simulink model "vehicle_motion_model_final_temp"  (R2021b)
settings: Solver=ode5  StartTime=0.0  StopTime=600  FixedStep=0.001  RelTol=1e-3
StopFcn:
  | % stop simulation callback function
  | figure(1);
  | out.x_gt.data = permute(out.x_gt.data,[3, 1, 2]);
  | plot3(out.x_gt.data(:, 1), out.x_gt.data(:, 2), -out.x_gt.data(:, 3), 'Color', 'r', 'LineWidth', 1.5);
  | legend('Истинная траектория')
  | xlabel('X, \itм');
  | ylabel('Y, \itм');
  | zlabel('Z, \itм');
  | figure(2);
  | plot3(out.x.data(:, 1), out.x.data(:, 2), -out.x.data(:, 3), 'Color', 'b', 'LineWidth', 1.5);
  | hold on;
  | xlabel('X, \itм');
  | ylabel('Y, \itм');
  | zlabel('Z, \itм');
  | % legend('pos')
  | hold on;
  | plot3(out.x_gt.data(:, 1), out.x_gt.data(:, 2), -out.x_gt.data(:, 3), 'Color', 'r', 'LineWidth', 1.5);
  | hold on;
  | legend('Рассчитанная траектория', 'Истинная траектория')
  | % errors
  | figure(3);
  | yyaxis left;
  | plot(out.hor_err_fus.time, out.hor_err_fus.data, 'Color', 'b', 'LineWidth', 1.5);
  | xlabel('время, \itс');
  | ylabel('Горизонтальная ошибка, \itм');
  | hold on;
  | yyaxis right;
  | plot(out.ver_err_fus.time, out.ver_err_fus.data, 'Color', 'r', 'LineWidth', 1.5);
  | ylabel('Вертикальная ошибка, \itм');
  | legend('Горизонтальная позиционная ошибка', 'Вертикальная позиционная ошибка');
  | grid on;
  | figure(4);
  | yyaxis left;
  | plot(out.hor_err_ins.time, out.hor_err_ins.data, '-', 'Color', 'b', 'LineWidth', 1.5);
  | xlabel('время, \itс');
  | ylabel('Горизонтальная ошибка, \itм');
  | hold on;
  | yyaxis right;
  | plot(out.ver_err_ins.time, out.ver_err_ins.data, '-', 'Color', 'r', 'LineWidth', 1.5);
  | ylabel('Вертикальная ошибка, \itм');
  | legend('Горизонтальная позиционная ошибка', 'Вертикальная позиционная ошибка');
  | grid on;
model workspace (MAT data in the model file):
  AxlIxx = 62.3745166667
  AxlM = 160
  Cps = 2
  CzWhlAxl = 557955.087061
  DCT_Param : object (value not decoded)
  Downshift_Speeds = [9.5625 12.9375 16.3125 19.6875 23.0625 26.4375 29.8125 33.1875 36.5625 39.9375 43.3125 46.6875 ... (28 elements, 4x7)]
  F0zWhlAxl = 16132.2380068
  HTCH : object (value not decoded)
  Hmax = 0.25
  KzWhlAxl = 58428920.0848
  NCyl = 6
  Pedal_Positions = [0.1 0.4 0.5 0.9]
  Pstd = 101325
  Q = [1  0  0; 0  1  0; 0  0  1]
  Rair = 287
  SUS : object (value not decoded)
  TRA : object (value not decoded)
  Trans : object (value not decoded)
  Tstd = 293.15
  Upshift_Speeds = [12.9375 16.3125 19.6875 33 26.4375 29.8125 33.1875 52.5 39.9375 43.3125 46.6875 77.25 ... (28 elements, 4x7)]
  VEH : object (value not decoded)
  Vd = 0.00346
  WH : Mass (value not decoded)
  dt3D = 0.05
  f_air = [0 0 0 0 0 0 0 0 0 0 0 0 ... (256 elements, 16x16)]
  f_co = [0 0 0 0 0 0 0 0 0 0 0 0 ... (256 elements, 16x16)]
  f_co2 = [0 0 0 0 0 0 0 0 0 0 0 0 ... (256 elements, 16x16)]
  f_eff = [352.135682859 352.135682859 320.724378192 303.655312657 295.930136708 291.240087194 291.240271258 291.240312459 291.240275452 291.240198499 291.240100781 291.240018769 ... (256 elements, 16x16)]
  f_fuel = [0 0 0 0 0 0 0 0 0 0 0 0 ... (256 elements, 16x16)]
  f_hc = [0 0 0 0 0 0 0 0 0 0 0 0 ... (256 elements, 16x16)]
  f_nox = [0 0 0 0 0 0 0 0 0 0 0 0 ... (256 elements, 16x16)]
  f_pm = [0 0 0 0 0 0 0 0 0 0 0 0 ... (256 elements, 16x16)]
  f_susp_axl_bp = [1 2]
  f_susp_dz_bp = [-0.325022776267 -0.315022776267 -0.305022776267 -0.205022776267 -0.105022776267 -0.00502277626717 0.0949772237328 0.194977223733 0.204977223733 0.214977223733]
  f_susp_dzdot_bp = [-3 -0.3 -0.2 -0.1 0 0.1 0.2 0.3 3]
  f_susp_fmz = [-144070.391448 -93629.24037 -75929.1118915 -20630.5828179 -15385.48216 -10140.3815021 -4895.28084414 349.819813785 -31916.3973792 18437.6709544 -83996.1993354 -33555.0482577 ... (43920 elements, 10x9x61x2x4)]
  f_susp_geom = [0 0 0 0 0 0 0 0 0 0 0 0 ... (3660 elements, 10x61x2x3)]
  f_susp_strgdelta_bp = [-0.523598775598 -0.506145483078 -0.488692190558 -0.471238898038 -0.453785605519 -0.436332312999 -0.418879020479 -0.401425727959 -0.383972435439 -0.366519142919 -0.349065850399 -0.331612557879 ... (61 elements, 1x61)]
  f_tbrake = [0 76.8593923996 105.140482948 131.533638111 157.926793274 176.658631717 176.65727296 176.656856686 176.656879077 176.657093756 176.657404516 176.65772406 ... (256 elements, 16x16)]
  f_tbrake_n_bpt = [0 649.519052838 912.419621844 1175.32019085 1438.22075986 1701.12132886 1964.02189787 2226.92246687 2489.82303588 2752.72360489 3015.62417389 3278.5247429 ... (16 elements, 1x16)]
  f_tbrake_t_bpt = [0 34.6410161514 61.0341713143 87.4273264773 113.82048164 140.213636803 166.606791966 192.999947129 219.393102292 245.786257455 272.179412618 298.572567781 ... (16 elements, 1x16)]
  f_texh = [766.752464599 766.752464599 786.17542386 801.679939032 884.591982581 910.574397722 910.571871054 910.570774534 910.570601632 910.570821151 910.571247242 910.571639815 ... (256 elements, 16x16)]
  f_twc_eff_co = [0.17 0.25 0.45 0.99 0.99 0.99 0.99]
  f_twc_eff_hc = [0.21 0.375 0.75 0.98 0.98 0.98 0.98]
  f_twc_eff_lam = [0.909090909 0.944055944 0.979020979 1 1.013986014 1.048951049 1.083916084]
  f_twc_eff_nox = [0.98 0.98 0.98 0.97 0.05 0.02 0]
  h = 0.134
symbols that are objects in the model workspace (value not decoded): VEH
libraries: aerolibcommonsys x8, sharedtransform x8, sharedutil x7, autolibsharedcommon x7, autolibutils x4, vehdynlibtirecommon x3, dspstat3 x2, mspsensorlib x1, aerolibnav x1, shared6dof x1, autolibshared x1, vehdynlibsuspension x1
(part 8 of 9)

== system vehicle_motion_model_final_temp/Two-Axle Vehicle/Wheels and Tires/Wheels and Tires/Veh2Tire/Wheel Angles ==
  steer : Inport
  camber : Inport  Port=2
  Add1 : Sum
  Add2 : Sum
  Constant1 : Constant  Value=pi
  Constant2 : Constant  Value=[pi;0;pi;0].*0+[0;pi;0;pi].*0
  Constant3 : Constant  Value=ones(1,4).*0
  Reshape : Reshape  OutputDimensionality=Row vector (2-D)
  Reshape1 : Reshape  OutputDimensionality=Row vector (2-D)
  Reshape2 : Reshape  OutputDimensionality=Row vector (2-D)
  Vector Concatenate3 : Concatenate  NumInputs=3  Mode=Multidimensional array
  Vehicle : Outport  VectorParamsAs1DForOutWhenUnconnected=off
  wires:
  Constant2/1 -> Add1/2
  Constant3/1 -> Reshape2/1
  Vector Concatenate3/1 -> Vehicle/1
  Reshape/1 -> Vector Concatenate3/3
  Reshape1/1 -> Vector Concatenate3/1
  camber/1 -> Add2/1
  Reshape2/1 -> Vector Concatenate3/2
  steer/1 -> Add1/1
  Add1/1 -> Reshape/1
  Constant1/1 -> Add2/2
  Add2/1 -> Reshape1/1

== system vehicle_motion_model_final_temp/Two-Axle Vehicle/Wheels and Tires/Wheels and Tires/Veh2Tire/Wheel to Body Transform ==
  VelVeh : Inport  Partition=on  PartitionDimension=2  PartitionWidth=1  PartitionOffset=0
  WheelAngles : Inport  Port=2  Partition=on  PartitionDimension=2  PartitionWidth=1  PartitionOffset=0
  Demux1 : Demux  Outputs=3
  Divide1 : Product  Inputs=**  Multiplication=Matrix(*)
  For Each : ForEach  DisableCoverage=on
  Rotation Angles to Direction Cosine Matrix : sharedtransform/Rotation Angles to Direction Cosine Matrix  rotationOrder=ZYX  aMode=2
      settings: SourceProductBaseCode=AE,PW,DR,MT,UV,VE
  Selector : Selector  InputPortWidth=3  IndexOptions=Index vector (dialog)  Indices=[3 2 1]  OutputSizes=1
  xdotWheel : Outport  ConcatenationDimension=1  VectorParamsAs1DForOutWhenUnconnected=off
  ydotWheel : Outport  Port=2  ConcatenationDimension=1  VectorParamsAs1DForOutWhenUnconnected=off
  zdotWheel : Outport  Port=3  ConcatenationDimension=1  VectorParamsAs1DForOutWhenUnconnected=off
  wires:
  Divide1/1 -> Demux1/1
  Demux1/1 -> xdotWheel/1
  Demux1/2 -> ydotWheel/1
  Demux1/3 -> zdotWheel/1
  Rotation Angles to Direction Cosine Matrix/1 -> Divide1/1
  VelVeh/1 -> Divide1/2
  WheelAngles/1 -> Selector/1
  Selector/1 -> Rotation Angles to Direction Cosine Matrix/1

== system vehicle_motion_model_final_temp/Two-Axle Vehicle/Vehicle Body/Vehicle Body 6DOF/Vehicle Body 6DOF/6 DOF Generic Vehicle Body/Aero Drag ==
  Body Vel : Inport
  DCM : Inport  Port=2
  Wind : Inport  Port=3
  Temp : Inport  Port=4  Unit=K
  Drag Force : autolibsharedcommon/Vehicle Body 3dof/Drag Force  A=Af  beta_w=beta_w  Cd=Cd  Cs=Cs  Cl=Cl  Cpm=Cpm  Lcpm=a+b  Crm=beta_w.*eps  Cym=Cym  R=287.058  Pabs=Pabs
      settings: SourceProductBaseCode=PW,DR,MT,UV,VE
  Inertial to Body : Product  Multiplication=Matrix(*)  InputSameDT=on  SaturateOnIntegerOverflow=on  OutDataTypeStr=Inherit: Same as first input
  Reshape1 : Reshape
  F : Outport  VectorParamsAs1DForOutWhenUnconnected=off
  M : Outport  Port=2  VectorParamsAs1DForOutWhenUnconnected=off
  wires:
  Temp/1 -> Drag Force/3
  Wind/1 -> Reshape1/1
  DCM/1 -> Inertial to Body/1
  Reshape1/1 -> Inertial to Body/2
  Drag Force/2 -> M/1
  Drag Force/1 -> F/1
  Inertial to Body/1 -> Drag Force/2
  Body Vel/1 -> Drag Force/1

== system vehicle_motion_model_final_temp/Two-Axle Vehicle/Vehicle Body/Vehicle Body 6DOF/Vehicle Body 6DOF/6 DOF Generic Vehicle Body/Gravity ==
  DCM : Inport
  Mbar : Inport  Port=2
  0 : Constant  Value=0
  Inertial to Body : Product  Multiplication=Matrix(*)  InputSameDT=on  SaturateOnIntegerOverflow=on  OutDataTypeStr=Inherit: Same as first input
  Product : Product
  Reshape : Reshape
  Vector Concatenate : Concatenate  NumInputs=3
  g : Constant  Value=g
  Fg : Outport  VectorParamsAs1DForOutWhenUnconnected=off
  wires:
  0/1 -> Vector Concatenate/1, Vector Concatenate/2
  Vector Concatenate/1 -> Product/1  "Inertial gravity vector"
  Mbar/1 -> Product/2
  Inertial to Body/1 -> Fg/1  "Fg_B"
  g/1 -> Vector Concatenate/3
  Reshape/1 -> Inertial to Body/2
  Product/1 -> Reshape/1  "Fg_I"
  DCM/1 -> Inertial to Body/1

== system vehicle_motion_model_final_temp/Two-Axle Vehicle/Vehicle Body/Vehicle Body 6DOF/Vehicle Body 6DOF/6 DOF Generic Vehicle Body/Power Calculations ==
  FBody : Inport
  Fdrag : Inport  Port=2
  v : Inport  Port=3
  Mdrag : Inport  Port=4
  Mtotal : Inport  Port=5
  p,q,r : Inport  Port=6
  Abs : Abs  ZeroCross=off
  Abs1 : Abs  ZeroCross=off
  Bus Creator1 : BusCreator  Inputs=2
  Product{1..2,8..9} (4 alike) : Product
  Signal Specification : SignalSpecification  Unit=W
  Signal Specification1 : SignalSpecification  Unit=W
  Sum of Elements : Sum  Inputs=+
  Sum of Elements1 : Sum  Inputs=+
  Vector Concatenate : Concatenate
  Vector Concatenate1 : Concatenate
  Pwr : Outport  VectorParamsAs1DForOutWhenUnconnected=off
  wires:
  v/1 -> Product9/1, Product8/2
  Vector Concatenate1/1 -> Abs1/1
  Vector Concatenate/1 -> Abs/1
  p,q,r/1 -> Product1/2, Product2/1
  Product2/1 -> Vector Concatenate1/2
  Product1/1 -> Vector Concatenate/2
  Mdrag/1 -> Product2/2
  Mtotal/1 -> Product1/1
  Sum of Elements1/1 -> Signal Specification/1
  Sum of Elements/1 -> Signal Specification1/1
  Abs1/1 -> Sum of Elements1/1
  Abs/1 -> Sum of Elements/1
  FBody/1 -> Product8/1
  Fdrag/1 -> Product9/2
  Product8/1 -> Vector Concatenate/1
  Signal Specification/1 -> Bus Creator1/2  "Drag"
  Signal Specification1/1 -> Bus Creator1/1  "PwrExt"
  Product9/1 -> Vector Concatenate1/1
  Bus Creator1/1 -> Pwr/1  "Pwr"

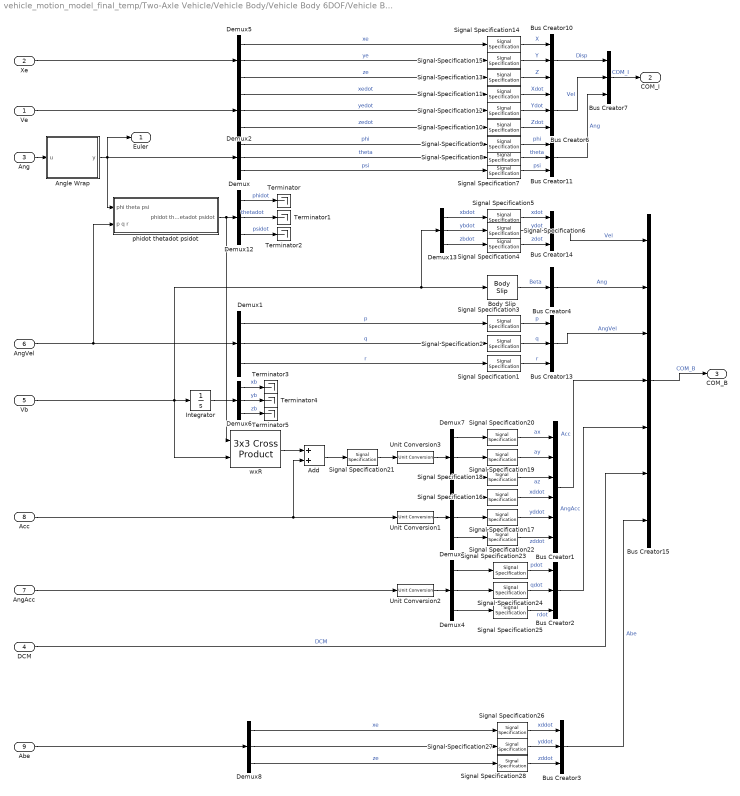
== system vehicle_motion_model_final_temp/Two-Axle Vehicle/Vehicle Body/Vehicle Body 6DOF/Vehicle Body 6DOF/6 DOF Generic Vehicle Body/SignalCollection ==
  Ve : Inport
  Xe : Inport  Port=2
  Ang : Inport  Port=3
  DCM : Inport  Port=4
  Vb : Inport  Port=5
  AngVel : Inport  Port=6
  AngAcc : Inport  Port=7
  Acc : Inport  Port=8
  Abe : Inport  Port=9
  Add : Sum
  Angle Wrap : Subsystem  Variant=on  VariantControlMode=label  VariantControl=Variant1  LabelModeActiveChoice=Unwrap
  Body Slip : autolibshared/Vehicle Body 3DOF Single Track/Signal Routing/Signal Routing/state2bus/Body Slip  mask{xdot_tol=xdot_tol}
      mask prompts: xdot_tol "Longituindal low speed tolerance, xdot_tol [m/s]:"
      settings: SourceProductBaseCode=PW,DR,MT,UV,VE
  Bus Creator1 : BusCreator  Inputs=6
  Bus Creator{2..3,6..7,10..11,13..14} (8 alike) : BusCreator  Inputs=3
  Bus Creator15 : BusCreator  Inputs=7
  Bus Creator4 : BusCreator  Inputs=1
  Demux{,1..8,12..13} (11 alike) : Demux  Outputs=3
  Integrator : Integrator
  Signal Specification1 : SignalSpecification  Unit=rad/s
  Signal Specification{4..6,10..12} (6 alike) : SignalSpecification  Unit=m/s
  Signal Specification13 : SignalSpecification  Unit=m
  Signal Specification14 : SignalSpecification  Unit=m
  Signal Specification15 : SignalSpecification  Unit=m
  Signal Specification{16..17,21..22,26..28} (7 alike) : SignalSpecification  Unit=m/s^2
  Signal Specification18 : SignalSpecification  Unit=gn
  Signal Specification19 : SignalSpecification  Unit=gn
  Signal Specification2 : SignalSpecification  Unit=rad/s
  Signal Specification20 : SignalSpecification  Unit=gn
  Signal Specification23 : SignalSpecification  Unit=rad/s^2
  Signal Specification24 : SignalSpecification  Unit=rad/s^2
  Signal Specification25 : SignalSpecification  Unit=rad/s^2
  Signal Specification3 : SignalSpecification  Unit=rad/s
  Signal Specification7 : SignalSpecification  Unit=rad
  Signal Specification8 : SignalSpecification  Unit=rad
  Signal Specification9 : SignalSpecification  Unit=rad
  Terminator{,1..5} (6 alike) : Terminator
  Unit Conversion1 : UnitConversion
  Unit Conversion2 : UnitConversion
  Unit Conversion3 : UnitConversion
  phidot thetadot psidot : Subsystem
  wxR : sharedutil/3x3 Cross Product  aMode=aMode
      settings: SourceProductBaseCode=AE,PW,DR,MT,UV,VE
  Euler : Outport  Unit=rad  VectorParamsAs1DForOutWhenUnconnected=off
  COM_I : Outport  Port=2  VectorParamsAs1DForOutWhenUnconnected=off
  COM_B : Outport  Port=3  VectorParamsAs1DForOutWhenUnconnected=off
  wires:
  Bus Creator3/1 -> Bus Creator15/7  "Abe"
  Signal Specification26/1 -> Bus Creator3/1  "xddot"
  Abe/1 -> Demux8/1
  Signal Specification27/1 -> Bus Creator3/2  "yddot"
  Signal Specification28/1 -> Bus Creator3/3  "zddot"
  Demux8/3 -> Signal Specification28/1  "ze"
  Demux8/2 -> Signal Specification27/1
  Demux8/1 -> Signal Specification26/1  "xe"
  Signal Specification24/1 -> Bus Creator2/2  "qdot"
  Signal Specification25/1 -> Bus Creator2/3  "rdot"
  Signal Specification23/1 -> Bus Creator2/1  "pdot"
  Bus Creator2/1 -> Bus Creator15/5  "AngAcc"
  Unit Conversion2/1 -> Demux4/1
  Angle Wrap/1(" y") -> Euler/1, Demux/1, phidot thetadot psidot/1(phi theta psi)
  Ve/1 -> Demux2/1
  Body Slip/1 -> Bus Creator4/1  "Beta"
  Bus Creator4/1 -> Bus Creator15/2  "Ang"
  DCM/1 -> Bus Creator15/6  "DCM"
  Signal Specification16/1 -> Bus Creator1/4  "xddot"
  Signal Specification22/1 -> Bus Creator1/6  "zddot"
  Signal Specification17/1 -> Bus Creator1/5  "yddot"
  Unit Conversion1/1 -> Demux3/1
  Signal Specification21/1 -> Unit Conversion3/1
  Unit Conversion3/1 -> Demux7/1
  Add/1 -> Signal Specification21/1
  Acc/1 -> Unit Conversion1/1, Add/2
  Demux7/3 -> Signal Specification18/1
  Demux7/1 -> Signal Specification20/1
  Demux7/2 -> Signal Specification19/1
  wxR/1 -> Add/1
  Signal Specification19/1 -> Bus Creator1/2  "ay"
  Signal Specification20/1 -> Bus Creator1/1  "ax"
  Signal Specification18/1 -> Bus Creator1/3  "az"
  Bus Creator1/1 -> Bus Creator15/4  "Acc"
  Bus Creator10/1 -> Bus Creator7/1  "Disp"
  Signal Specification14/1 -> Bus Creator10/1  "X"
  Signal Specification15/1 -> Bus Creator10/2  "Y"
  Bus Creator14/1 -> Bus Creator15/1  "Vel"
  Signal Specification10/1 -> Bus Creator6/3  "Zdot"
  Signal Specification12/1 -> Bus Creator6/2  "Ydot"
  Signal Specification2/1 -> Bus Creator13/2  "q"
  Signal Specification13/1 -> Bus Creator10/3  "Z"
  Signal Specification5/1 -> Bus Creator14/1  "xdot"
  Signal Specification11/1 -> Bus Creator6/1  "Xdot"
  Bus Creator15/1 -> COM_B/1  "COM_B"
  Signal Specification8/1 -> Bus Creator11/2  "theta"
  Bus Creator6/1 -> Bus Creator7/2  "Vel"
  Signal Specification4/1 -> Bus Creator14/3  "zdot"
  Bus Creator11/1 -> Bus Creator7/3  "Ang"
  Signal Specification7/1 -> Bus Creator11/3  "psi"
  Signal Specification6/1 -> Bus Creator14/2  "ydot"
  Signal Specification1/1 -> Bus Creator13/3  "r"
  Signal Specification3/1 -> Bus Creator13/1  "p"
  Bus Creator13/1 -> Bus Creator15/3  "AngVel"
  Signal Specification9/1 -> Bus Creator11/1  "phi"
  Demux6/3 -> Terminator5/1  "zb"
  Demux6/2 -> Terminator4/1  "yb"
  Demux6/1 -> Terminator3/1  "xb"
  Integrator/1 -> Demux6/1
  Demux1/1 -> Signal Specification3/1  "p"
  Bus Creator7/1 -> COM_I/1  "COM_I"
  Vb/1 -> Integrator/1, Body Slip/1, Demux13/1, wxR/2
  Demux13/3 -> Signal Specification4/1  "zbdot"
  Demux13/2 -> Signal Specification6/1  "ybdot"
  Demux13/1 -> Signal Specification5/1  "xbdot"
  AngVel/1 -> Demux1/1, phidot thetadot psidot/2(p q r)
  phidot thetadot psidot/1(phidot thetadot psidot) -> Demux12/1, wxR/1
  Demux12/3 -> Terminator2/1  "psidot"
  Demux12/2 -> Terminator1/1  "thetadot"
  Demux12/1 -> Terminator/1  "phidot"
  Ang/1 -> Angle Wrap/1("u ")
  Demux4/3 -> Signal Specification25/1
  Demux4/2 -> Signal Specification24/1
  Demux4/1 -> Signal Specification23/1
  Demux5/3 -> Signal Specification13/1  "ze"
  Demux5/2 -> Signal Specification15/1  "ye"
  Demux5/1 -> Signal Specification14/1  "xe"
  Xe/1 -> Demux5/1
  Demux3/3 -> Signal Specification22/1
  Demux3/2 -> Signal Specification17/1
  Demux3/1 -> Signal Specification16/1
  Demux2/3 -> Signal Specification10/1  "zedot"
  Demux2/2 -> Signal Specification12/1  "yedot"
  Demux2/1 -> Signal Specification11/1  "xedot"
  Demux1/3 -> Signal Specification1/1  "r"
  Demux1/2 -> Signal Specification2/1  "q"
  Demux/3 -> Signal Specification7/1  "psi"
  Demux/2 -> Signal Specification8/1  "theta"
  Demux/1 -> Signal Specification9/1  "phi"
  AngAcc/1 -> Unit Conversion2/1

== system vehicle_motion_model_final_temp/Two-Axle Vehicle/Vehicle Body/Vehicle Body 6DOF/Vehicle Body 6DOF/6 DOF Generic Vehicle Body/Wheel to CG ==
  MSusp : Inport
  Selector1 : Selector  NumberOfDimensions=2  InputPortWidth=3  IndexOptions=Index vector (dialog),Select all  Indices=[1],1  OutputSizes=1,1
  Selector2 : Selector  NumberOfDimensions=2  InputPortWidth=3  IndexOptions=Index vector (dialog),Select all  Indices=[2],1  OutputSizes=1,1
  Selector3 : Selector  NumberOfDimensions=2  InputPortWidth=3  IndexOptions=Index vector (dialog),Select all  Indices=[3],1  OutputSizes=1,1
  Sum of Elements : Sum  Inputs=+
  Sum of Elements1 : Sum  Inputs=+
  Sum of Elements2 : Sum  Inputs=+
  Vector Concatenate : Concatenate  NumInputs=3
  MVeh : Outport  VectorParamsAs1DForOutWhenUnconnected=off
  wires:
  Selector3/1 -> Sum of Elements2/1
  Selector1/1 -> Sum of Elements/1
  Selector2/1 -> Sum of Elements1/1
  MSusp/1 -> Selector1/1, Selector2/1, Selector3/1
  Vector Concatenate/1 -> MVeh/1
  Sum of Elements2/1 -> Vector Concatenate/3
  Sum of Elements1/1 -> Vector Concatenate/2
  Sum of Elements/1 -> Vector Concatenate/1

== system vehicle_motion_model_final_temp/Two-Axle Vehicle/Vehicle Body/Vehicle Body 6DOF/Vehicle Body 6DOF/Moment Calc/Hitch moments from forces ==
  Rbar : Inport
  Fh : Inport  Port=2
  Constant : Constant  Value=d
  Constant1 : Constant  Value=h
  Demux : Demux  Outputs=3
  Demux1 : Demux  Outputs=3
  Mux : Mux  Inputs=3
  Mx : Sum  Inputs=-+
  My : Sum
  Mz : Sum  Inputs=--
  Product{,1..5} (6 alike) : Product
  Sum1 : Sum  Inputs=+--
  Sum3 : Sum  Inputs=+--
  Sum4 : Sum
  hitch geometry parameters : Subsystem  Variant=on  VariantControlMode=label  LabelModeActiveChoice=0
  Mroll : Outport  VectorParamsAs1DForOutWhenUnconnected=off
  Mpitch : Outport  Port=2  VectorParamsAs1DForOutWhenUnconnected=off
  Myaw : Outport  Port=3  VectorParamsAs1DForOutWhenUnconnected=off
  Hbar : Outport  Port=4  VectorParamsAs1DForOutWhenUnconnected=off
  wires:
  Mux/1 -> Hbar/1
  Product5/1 -> Mx/2
  Product4/1 -> Mx/1
  Product3/1 -> My/2
  Demux1/3 -> Product3/1, Product5/2
  Product2/1 -> Mz/2
  Sum4/1 -> Product3/2, Product2/2, Mux/1
  Demux1/2 -> Product2/1, Product4/2
  Mx/1 -> Mroll/1
  Sum3/1 -> Product1/2, Product5/1, Mux/2
  Product1/1 -> Mz/1
  Mz/1 -> Myaw/1
  My/1 -> Mpitch/1
  Product/1 -> My/1
  Sum1/1 -> Product/1, Product4/1, Mux/3
  Demux1/1 -> Product/2, Product1/1
  Fh/1 -> Demux1/1
  Constant1/1 -> Sum1/1
  Constant/1 -> Sum3/2
  hitch geometry parameters/1(dh_out) -> Sum4/1
  Demux/1 -> Sum4/2
  Rbar/1 -> Demux/1
  Demux/3 -> Sum1/2
  Demux/2 -> Sum3/3
  hitch geometry parameters/3(hh_out) -> Sum1/3
  hitch geometry parameters/2(hl_out) -> Sum3/1

== system vehicle_motion_model_final_temp/Two-Axle Vehicle/Vehicle Body/Vehicle Body 6DOF/Vehicle Body 6DOF/Signal Routing/Hard Point Coordinate Transform Front Left ==
  InertFrmCg : Inport
  BdyFrmCg : Inport  Port=2
  HPbar : Inport  Port=3
  Hard Point Coordinate Transform External Displacement : autolibsharedcommon/Hard Point Coordinate Transform External Displacement  aMode=aMode
      settings: SourceProductBaseCode=PW,DR,MT,UV,VE
  Selector1 : Selector  NumberOfDimensions=2  InputPortWidth=3  IndexOptions=Select all,Index vector (dialog)  Indices=[1],[1]  OutputSizes=1,1
  Inert : Outport  VectorParamsAs1DForOutWhenUnconnected=off
  Body : Outport  Port=2  VectorParamsAs1DForOutWhenUnconnected=off
  wires:
  HPbar/1 -> Selector1/1
  Hard Point Coordinate Transform External Displacement/1 -> Inert/1
  BdyFrmCg/1 -> Hard Point Coordinate Transform External Displacement/2
  Selector1/1 -> Hard Point Coordinate Transform External Displacement/3
  Hard Point Coordinate Transform External Displacement/2 -> Body/1
  InertFrmCg/1 -> Hard Point Coordinate Transform External Displacement/1

== system vehicle_motion_model_final_temp/Two-Axle Vehicle/Vehicle Body/Vehicle Body 6DOF/Vehicle Body 6DOF/Signal Routing/Hard Point Coordinate Transform Front Right ==
  InertFrmCg : Inport
  BdyFrmCg : Inport  Port=2
  HPbar : Inport  Port=3
  Hard Point Coordinate Transform External Displacement : autolibsharedcommon/Hard Point Coordinate Transform External Displacement  aMode=aMode
      settings: SourceProductBaseCode=PW,DR,MT,UV,VE
  Selector1 : Selector  NumberOfDimensions=2  InputPortWidth=3  IndexOptions=Select all,Index vector (dialog)  Indices=[1],[2]  OutputSizes=1,1
  Inert : Outport  VectorParamsAs1DForOutWhenUnconnected=off
  Body : Outport  Port=2  VectorParamsAs1DForOutWhenUnconnected=off
  wires:
  Selector1/1 -> Hard Point Coordinate Transform External Displacement/3
  HPbar/1 -> Selector1/1
  InertFrmCg/1 -> Hard Point Coordinate Transform External Displacement/1
  Hard Point Coordinate Transform External Displacement/2 -> Body/1
  BdyFrmCg/1 -> Hard Point Coordinate Transform External Displacement/2
  Hard Point Coordinate Transform External Displacement/1 -> Inert/1

== system vehicle_motion_model_final_temp/Two-Axle Vehicle/Vehicle Body/Vehicle Body 6DOF/Vehicle Body 6DOF/Signal Routing/Hard Point Coordinate Transform Geometric ==
  InertFrmCg : Inport
  BdyFrmCg : Inport  Port=2
  Rbar : Inport  Port=3
  Hard Point Coordinate Transform External Displacement Beta : autolibsharedcommon/Hard Point Coordinate Transform External Displacement Beta  xdot_tol=xdot_tol  aMode=aMode
      settings: SourceProductBaseCode=PW,DR,MT,UV,VE
  Subtract : Sum
  Vector Concatenate : Concatenate  NumInputs=3
  latOff : Constant  Value=latOff
  longOff : Constant  Value=longOff
  "vertOff " : Constant  Value=vertOff
  Inert : Outport  VectorParamsAs1DForOutWhenUnconnected=off
  Body : Outport  Port=2  VectorParamsAs1DForOutWhenUnconnected=off
  wires:
  Subtract/1 -> Hard Point Coordinate Transform External Displacement Beta/3
  Rbar/1 -> Subtract/2
  latOff/1 -> Vector Concatenate/2
  longOff/1 -> Vector Concatenate/1
  "vertOff "/1 -> Vector Concatenate/3
  Hard Point Coordinate Transform External Displacement Beta/1 -> Inert/1
  BdyFrmCg/1 -> Hard Point Coordinate Transform External Displacement Beta/2
  Vector Concatenate/1 -> Subtract/1
  Hard Point Coordinate Transform External Displacement Beta/2 -> Body/1
  InertFrmCg/1 -> Hard Point Coordinate Transform External Displacement Beta/1

== system vehicle_motion_model_final_temp/Two-Axle Vehicle/Vehicle Body/Vehicle Body 6DOF/Vehicle Body 6DOF/Signal Routing/Hard Point Coordinate Transform Hitch ==
  InertFrmCg : Inport
  BdyFrmCg : Inport  Port=2
  Hbar : Inport  Port=3
  Demux : Demux  Outputs=3
  Hard Point Coordinate Transform External Displacement : autolibsharedcommon/Hard Point Coordinate Transform External Displacement  aMode=aMode
      settings: SourceProductBaseCode=PW,DR,MT,UV,VE
  Unary Minus2 : UnaryMinus
  Vector Concatenate : Concatenate  NumInputs=3
  Inert : Outport  VectorParamsAs1DForOutWhenUnconnected=off
  Body : Outport  Port=2  VectorParamsAs1DForOutWhenUnconnected=off
  wires:
  Vector Concatenate/1 -> Hard Point Coordinate Transform External Displacement/3
  Demux/3 -> Vector Concatenate/3
  Demux/2 -> Vector Concatenate/2
  Demux/1 -> Unary Minus2/1
  Hbar/1 -> Demux/1
  Unary Minus2/1 -> Vector Concatenate/1
  Hard Point Coordinate Transform External Displacement/1 -> Inert/1
  BdyFrmCg/1 -> Hard Point Coordinate Transform External Displacement/2
  Hard Point Coordinate Transform External Displacement/2 -> Body/1
  InertFrmCg/1 -> Hard Point Coordinate Transform External Displacement/1

== system vehicle_motion_model_final_temp/Two-Axle Vehicle/Vehicle Body/Vehicle Body 6DOF/Vehicle Body 6DOF/Signal Routing/Hard Point Coordinate Transform Rear Left ==
  InertFrmCg : Inport
  BdyFrmCg : Inport  Port=2
  HPbar : Inport  Port=3
  Hard Point Coordinate Transform External Displacement : autolibsharedcommon/Hard Point Coordinate Transform External Displacement  aMode=aMode
      settings: SourceProductBaseCode=PW,DR,MT,UV,VE
  Selector1 : Selector  NumberOfDimensions=2  InputPortWidth=3  IndexOptions=Select all,Index vector (dialog)  Indices=[1],[3]  OutputSizes=1,1
  Inert : Outport  VectorParamsAs1DForOutWhenUnconnected=off
  Body : Outport  Port=2  VectorParamsAs1DForOutWhenUnconnected=off
  wires:
  Selector1/1 -> Hard Point Coordinate Transform External Displacement/3
  HPbar/1 -> Selector1/1
  Hard Point Coordinate Transform External Displacement/1 -> Inert/1
  BdyFrmCg/1 -> Hard Point Coordinate Transform External Displacement/2
  Hard Point Coordinate Transform External Displacement/2 -> Body/1
  InertFrmCg/1 -> Hard Point Coordinate Transform External Displacement/1

== system vehicle_motion_model_final_temp/Two-Axle Vehicle/Vehicle Body/Vehicle Body 6DOF/Vehicle Body 6DOF/Signal Routing/Hard Point Coordinate Transform Rear Right ==
  InertFrmCg : Inport
  BdyFrmCg : Inport  Port=2
  HPbar : Inport  Port=3
  Hard Point Coordinate Transform External Displacement : autolibsharedcommon/Hard Point Coordinate Transform External Displacement  aMode=aMode
      settings: SourceProductBaseCode=PW,DR,MT,UV,VE
  Selector1 : Selector  NumberOfDimensions=2  InputPortWidth=3  IndexOptions=Select all,Index vector (dialog)  Indices=[1],[4]  OutputSizes=1,1
  Inert : Outport  VectorParamsAs1DForOutWhenUnconnected=off
  Body : Outport  Port=2  VectorParamsAs1DForOutWhenUnconnected=off
  wires:
  Selector1/1 -> Hard Point Coordinate Transform External Displacement/3
  HPbar/1 -> Selector1/1
  InertFrmCg/1 -> Hard Point Coordinate Transform External Displacement/1
  Hard Point Coordinate Transform External Displacement/2 -> Body/1
  BdyFrmCg/1 -> Hard Point Coordinate Transform External Displacement/2
  Hard Point Coordinate Transform External Displacement/1 -> Inert/1

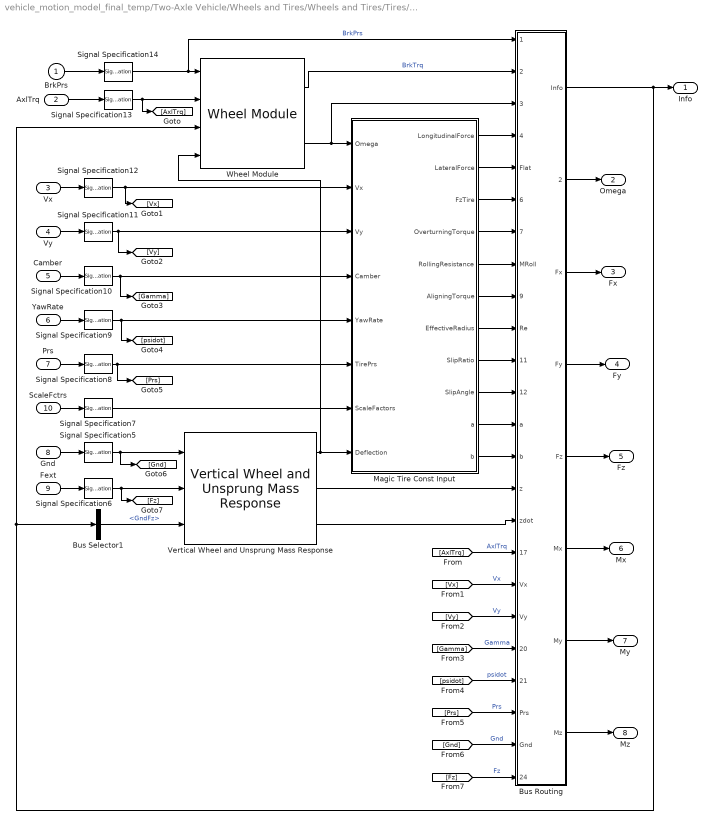
== system vehicle_motion_model_final_temp/Two-Axle Vehicle/Wheels and Tires/Wheels and Tires/Tires/MF Tires/Combined Slip Wheel 2DOF ==
  BrkPrs : Inport
  AxlTrq : Inport  Port=2
  Vx : Inport  Port=3
  Vy : Inport  Port=4
  Camber : Inport  Port=5
  YawRate : Inport  Port=6
  Prs : Inport  Port=7
  Gnd : Inport  Port=8
  Fext : Inport  Port=9
  ScaleFctrs : Inport  Port=10
  Bus Selector1 : BusSelector  OutputSignals=GndFz
  Bus Routing : Subsystem
  Magic Tire Const Input : Subsystem  AncestorBlock=vehdynlibtirecommon/Magic Tire Const Input
  Signal Specification10 : SignalSpecification  Unit=rad
  Signal Specification11 : SignalSpecification  Unit=m/s
  Signal Specification12 : SignalSpecification  Unit=m/s
  Signal Specification13 : SignalSpecification  Unit=N*m
  Signal Specification14 : SignalSpecification  Unit=Pa
  Signal Specification5 : SignalSpecification  Unit=m
  Signal Specification6 : SignalSpecification  Unit=N
  Signal Specification7 : SignalSpecification  Unit=1
  Signal Specification8 : SignalSpecification  Unit=Pa
  Signal Specification9 : SignalSpecification  Unit=rad/s
  Vertical Wheel and Unsprung Mass Response : vehdynlibtirecommon/Vertical Wheel and Unsprung Mass Response  m=MASS  bz=VERTICAL_DAMPING  zo=zo  zdoto=zdoto  g=GRAVITY  ReMax=UNLOADED_RADIUS
      settings: SourceProductBaseCode=VE
  Wheel Module : vehdynlibtirecommon/Wheel Module  Iyy=IYY
      settings: SourceProductBaseCode=VE
  Info : Outport  VectorParamsAs1DForOutWhenUnconnected=off
  Omega : Outport  Port=2  Unit=rad/s  VectorParamsAs1DForOutWhenUnconnected=off
  Fx : Outport  Port=3  Unit=N  VectorParamsAs1DForOutWhenUnconnected=off
  Fy : Outport  Port=4  Unit=N  VectorParamsAs1DForOutWhenUnconnected=off
  Fz : Outport  Port=5  Unit=N  VectorParamsAs1DForOutWhenUnconnected=off
  Mx : Outport  Port=6  Unit=N*m  VectorParamsAs1DForOutWhenUnconnected=off
  My : Outport  Port=7  Unit=N*m  VectorParamsAs1DForOutWhenUnconnected=off
  Mz : Outport  Port=8  Unit=N*m  VectorParamsAs1DForOutWhenUnconnected=off
  wires:
  [Fz] -> Bus Routing/24(FNormal)  "Fz"
  [Gnd] -> Bus Routing/23(Gnd)  "Gnd"
  [Prs] -> Bus Routing/22(Prs)  "Prs"
  [psidot] -> Bus Routing/21(psidot)  "psidot"
  [Gamma] -> Bus Routing/20(Gamma)  "Gamma"
  [Vy] -> Bus Routing/19(Vy)  "Vy"
  [Vx] -> Bus Routing/18(Vx)  "Vx"
  [AxlTrq] -> Bus Routing/17(AxlTrq)  "AxlTrq"
  Bus Routing/8(Mz) -> Mz/1
  Bus Routing/7(My) -> My/1
  Bus Routing/6(Mx) -> Mx/1
  Bus Routing/5(Fz) -> Fz/1
  Bus Routing/4(Fy) -> Fy/1
  Bus Routing/3(Fx) -> Fx/1
  Bus Routing/2(Omega) -> Omega/1
  Vertical Wheel and Unsprung Mass Response/3 -> Bus Routing/16(zdot)
  Vertical Wheel and Unsprung Mass Response/2 -> Bus Routing/15(z)
  Magic Tire Const Input/11(b) -> Bus Routing/14(b)
  Magic Tire Const Input/10(a) -> Bus Routing/13(a)
  Magic Tire Const Input/9(SlipAngle) -> Bus Routing/12(Alpha)
  Magic Tire Const Input/8(SlipRatio) -> Bus Routing/11(Kappa)
  Magic Tire Const Input/7(EffectiveRadius) -> Bus Routing/10(Re)
  Magic Tire Const Input/6(AligningTorque) -> Bus Routing/9(MAlign)
  Magic Tire Const Input/5(RollingResistance) -> Bus Routing/8(MRoll)
  Magic Tire Const Input/4(OverturningTorque) -> Bus Routing/7(MOver)
  Magic Tire Const Input/3(FzTire) -> Bus Routing/6(FzTire)
  Magic Tire Const Input/2(LateralForce) -> Bus Routing/5(Flat)
  Magic Tire Const Input/1(LongitudinalForce) -> Bus Routing/4(FLong)
  Bus Routing/1(Info) -> Info/1, Wheel Module/3, Bus Selector1/1
  BrkPrs/1 -> Signal Specification14/1
  Bus Selector1/1 -> Vertical Wheel and Unsprung Mass Response/3  "<GndFz>"
  Signal Specification14/1 -> Wheel Module/1, Bus Routing/1(BrkPrs)  "BrkPrs"
  AxlTrq/1 -> Signal Specification13/1
  Signal Specification13/1 -> Wheel Module/2, [AxlTrq]
  Signal Specification12/1 -> Magic Tire Const Input/2(Vx), [Vx]
  Vx/1 -> Signal Specification12/1
  Vy/1 -> Signal Specification11/1
  Signal Specification11/1 -> Magic Tire Const Input/3(Vy), [Vy]
  Camber/1 -> Signal Specification10/1
  Signal Specification10/1 -> Magic Tire Const Input/4(Camber), [Gamma]
  ScaleFctrs/1 -> Signal Specification7/1
  Signal Specification9/1 -> Magic Tire Const Input/5(YawRate), [psidot]
  YawRate/1 -> Signal Specification9/1
  Signal Specification8/1 -> Magic Tire Const Input/6(TirePrs), [Prs]
  Prs/1 -> Signal Specification8/1
  Signal Specification7/1 -> Magic Tire Const Input/7(ScaleFactors)
  Signal Specification6/1 -> Vertical Wheel and Unsprung Mass Response/2, [Fz]
  Fext/1 -> Signal Specification6/1
  Gnd/1 -> Signal Specification5/1
  Signal Specification5/1 -> Vertical Wheel and Unsprung Mass Response/1, [Gnd]
  Wheel Module/2 -> Bus Routing/3(omega), Magic Tire Const Input/1(Omega)
  Vertical Wheel and Unsprung Mass Response/1 -> Wheel Module/4, Magic Tire Const Input/8(Deflection)
  Wheel Module/1 -> Bus Routing/2(BrkTrq)  "BrkTrq"

== system vehicle_motion_model_final_temp/Two-Axle Vehicle/Vehicle Body/Vehicle Body 6DOF/Vehicle Body 6DOF/6 DOF Generic Vehicle Body/SignalCollection/Angle Wrap ==
  "u " : Inport
  None : Subsystem  VariantControl=None
  Unwrap : autolibutils/Unwrap  VariantControl=Unwrap  aMode=aMode
      settings: SourceProductBaseCode=PW,DR,MT,UV,VE
  " y" : Outport  VectorParamsAs1DForOutWhenUnconnected=off

== system vehicle_motion_model_final_temp/Two-Axle Vehicle/Vehicle Body/Vehicle Body 6DOF/Vehicle Body 6DOF/6 DOF Generic Vehicle Body/SignalCollection/phidot thetadot psidot ==
  phi theta psi : Inport
  p q r : Inport  Port=2
  Mux1 : Mux  Inputs=[3 3 3]
  Mux2 : Mux  Inputs=3
  phidot : Fcn  Expr=u[1]+(u[2]*u[4]+u[3]*u[7])*(u[5]/u[8])
  psidot : Fcn  Expr=(u[2]*u[4]+u[3]*u[7])/u[8]
  sincos : Trigonometry  Operator=sincos
  thetadot : Fcn  Expr=u[2]*u[7]-u[3]*u[4]
  phidot thetadot psidot : Outport  InitialOutput=0  VectorParamsAs1DForOutWhenUnconnected=off
  wires:
  sincos/2 -> Mux1/3
  sincos/1 -> Mux1/2
  Mux2/1 -> phidot thetadot psidot/1
  phidot/1 -> Mux2/1
  thetadot/1 -> Mux2/2
  psidot/1 -> Mux2/3
  phi theta psi/1 -> sincos/1
  p q r/1 -> Mux1/1
  Mux1/1 -> thetadot/1, phidot/1, psidot/1

== system vehicle_motion_model_final_temp/Two-Axle Vehicle/Vehicle Body/Vehicle Body 6DOF/Vehicle Body 6DOF/Moment Calc/Hitch moments from forces/hitch geometry parameters ==
  note: 1) Add Subsystem or Model blocks as valid variant choices.
      | 2) You cannot connect blocks at this level. At simulation, connectivity is automatically
      | determined, based on the active variant and port name matching.
  hitch active : Subsystem  VariantControl=1
  hitch inactive : Subsystem  VariantControl=0
  dh_out : Outport  Unit=m  VectorParamsAs1DForOutWhenUnconnected=off
  hl_out : Outport  Port=2  Unit=m  VectorParamsAs1DForOutWhenUnconnected=off
  hh_out : Outport  Port=3  Unit=m  VectorParamsAs1DForOutWhenUnconnected=off

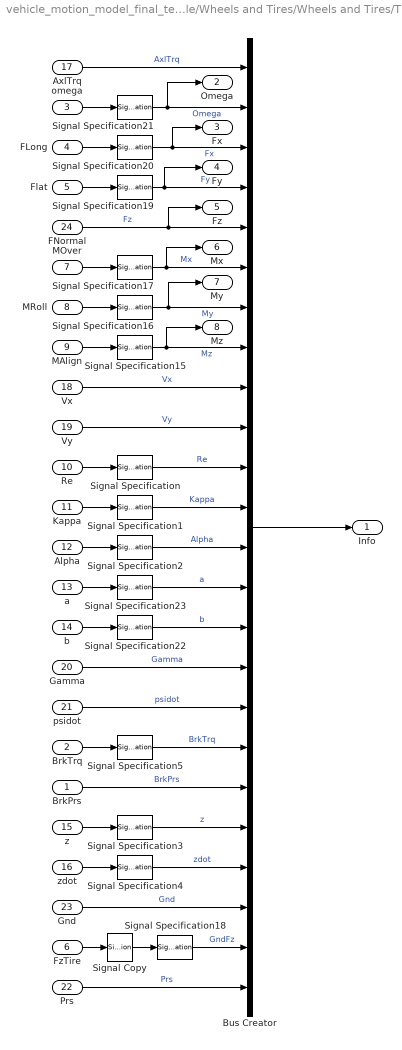
== system vehicle_motion_model_final_temp/Two-Axle Vehicle/Wheels and Tires/Wheels and Tires/Tires/MF Tires/Combined Slip Wheel 2DOF/Bus Routing ==
  BrkPrs : Inport
  BrkTrq : Inport  Port=2
  omega : Inport  Port=3
  FLong : Inport  Port=4
  Flat : Inport  Port=5
  FzTire : Inport  Port=6
  MOver : Inport  Port=7
  MRoll : Inport  Port=8
  MAlign : Inport  Port=9
  Re : Inport  Port=10
  Kappa : Inport  Port=11
  Alpha : Inport  Port=12
  a : Inport  Port=13
  b : Inport  Port=14
  z : Inport  Port=15
  zdot : Inport  Port=16
  AxlTrq : Inport  Port=17
  Vx : Inport  Port=18
  Vy : Inport  Port=19
  Gamma : Inport  Port=20
  psidot : Inport  Port=21
  Prs : Inport  Port=22
  Gnd : Inport  Port=23
  FNormal : Inport  Port=24
  Bus Creator : BusCreator  Inputs=24
  Signal Copy : SignalConversion  OverrideOpt=off
  Signal Specification{,3,22..23} (4 alike) : SignalSpecification  Unit=m
  Signal Specification1 : SignalSpecification  Unit=1
  Signal Specification{5,15..17} (4 alike) : SignalSpecification  Unit=N*m
  Signal Specification18 : SignalSpecification  Unit=N
  Signal Specification19 : SignalSpecification  Unit=N
  Signal Specification2 : SignalSpecification  Unit=rad
  Signal Specification20 : SignalSpecification  Unit=N
  Signal Specification21 : SignalSpecification  Unit=rad/s
  Signal Specification4 : SignalSpecification  Unit=m/s
  Info : Outport  VectorParamsAs1DForOutWhenUnconnected=off
  Omega : Outport  Port=2  Unit=rad/s  VectorParamsAs1DForOutWhenUnconnected=off
  Fx : Outport  Port=3  Unit=N  VectorParamsAs1DForOutWhenUnconnected=off
  Fy : Outport  Port=4  Unit=N  VectorParamsAs1DForOutWhenUnconnected=off
  Fz : Outport  Port=5  Unit=N  VectorParamsAs1DForOutWhenUnconnected=off
  Mx : Outport  Port=6  Unit=N*m  VectorParamsAs1DForOutWhenUnconnected=off
  My : Outport  Port=7  Unit=N*m  VectorParamsAs1DForOutWhenUnconnected=off
  Mz : Outport  Port=8  Unit=N*m  VectorParamsAs1DForOutWhenUnconnected=off
  wires:
  Signal Copy/1 -> Signal Specification18/1
  Prs/1 -> Bus Creator/24  "Prs"
  Gnd/1 -> Bus Creator/22  "Gnd"
  Signal Specification18/1 -> Bus Creator/23  "GndFz"
  BrkPrs/1 -> Bus Creator/19  "BrkPrs"
  Signal Specification5/1 -> Bus Creator/18  "BrkTrq"
  psidot/1 -> Bus Creator/17  "psidot"
  Gamma/1 -> Bus Creator/16  "Gamma"
  Vy/1 -> Bus Creator/10  "Vy"
  Vx/1 -> Bus Creator/9  "Vx"
  AxlTrq/1 -> Bus Creator/1  "AxlTrq"
  BrkTrq/1 -> Signal Specification5/1
  Kappa/1 -> Signal Specification1/1
  MRoll/1 -> Signal Specification16/1
  z/1 -> Signal Specification3/1
  zdot/1 -> Signal Specification4/1
  Re/1 -> Signal Specification/1
  b/1 -> Signal Specification22/1
  Flat/1 -> Signal Specification19/1
  MAlign/1 -> Signal Specification15/1
  FzTire/1 -> Signal Copy/1
  Signal Specification22/1 -> Bus Creator/15  "b"
  Signal Specification23/1 -> Bus Creator/14  "a"
  Signal Specification20/1 -> Fx/1, Bus Creator/3  "Fx"
  Signal Specification2/1 -> Bus Creator/13  "Alpha"
  omega/1 -> Signal Specification21/1
  Signal Specification16/1 -> My/1, Bus Creator/7  "My"
  Signal Specification19/1 -> Fy/1, Bus Creator/4  "Fy"
  FLong/1 -> Signal Specification20/1
  Signal Specification1/1 -> Bus Creator/12  "Kappa"
  MOver/1 -> Signal Specification17/1
  Signal Specification17/1 -> Bus Creator/6, Mx/1  "Mx"
  Bus Creator/1 -> Info/1
  Signal Specification/1 -> Bus Creator/11  "Re"
  Signal Specification15/1 -> Mz/1, Bus Creator/8  "Mz"
  FNormal/1 -> Fz/1, Bus Creator/5  "Fz"
  Signal Specification21/1 -> Omega/1, Bus Creator/2  "Omega"
  Signal Specification4/1 -> Bus Creator/21  "zdot"
  Alpha/1 -> Signal Specification2/1
  a/1 -> Signal Specification23/1
  Signal Specification3/1 -> Bus Creator/20  "z"

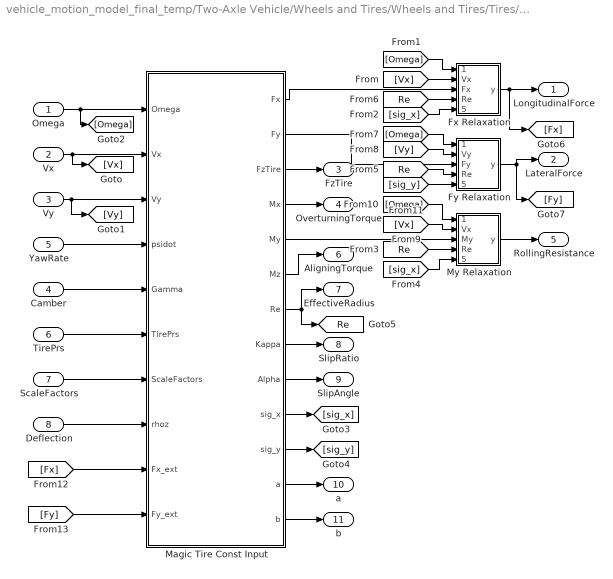
== system vehicle_motion_model_final_temp/Two-Axle Vehicle/Wheels and Tires/Wheels and Tires/Tires/MF Tires/Combined Slip Wheel 2DOF/Magic Tire Const Input ==
  Omega : Inport
  Vx : Inport  Port=2
  Vy : Inport  Port=3
  Camber : Inport  Port=4
  YawRate : Inport  Port=5
  TirePrs : Inport  Port=6
  ScaleFactors : Inport  Port=7
  Deflection : Inport  Port=8
  Fx Relaxation : Subsystem
  Fy Relaxation : Subsystem
  Magic Tire Const Input : MATLAB Function
  My Relaxation : Subsystem
  LongitudinalForce : Outport  VectorParamsAs1DForOutWhenUnconnected=off
  LateralForce : Outport  Port=2  VectorParamsAs1DForOutWhenUnconnected=off
  FzTire : Outport  Port=3  VectorParamsAs1DForOutWhenUnconnected=off
  OverturningTorque : Outport  Port=4  VectorParamsAs1DForOutWhenUnconnected=off
  RollingResistance : Outport  Port=5  VectorParamsAs1DForOutWhenUnconnected=off
  AligningTorque : Outport  Port=6  VectorParamsAs1DForOutWhenUnconnected=off
  EffectiveRadius : Outport  Port=7  VectorParamsAs1DForOutWhenUnconnected=off
  SlipRatio : Outport  Port=8  VectorParamsAs1DForOutWhenUnconnected=off
  SlipAngle : Outport  Port=9  VectorParamsAs1DForOutWhenUnconnected=off
  a : Outport  Port=10  VectorParamsAs1DForOutWhenUnconnected=off
  b : Outport  Port=11  VectorParamsAs1DForOutWhenUnconnected=off
  tag scope: Re=global
  wires:
  [Fy] -> Magic Tire Const Input/10(Fy_ext)
  [Fx] -> Magic Tire Const Input/9(Fx_ext)
  Magic Tire Const Input/1(Fx) -> Fx Relaxation/3(Fx)
  [sig_y] -> Fy Relaxation/5(sig_y)
  [Omega] -> My Relaxation/1(omega)
  [Vx] -> My Relaxation/2(Vx)
  [Vy] -> Fy Relaxation/2(Vy)
  [Omega] -> Fy Relaxation/1(omega)
  [Re] -> Fx Relaxation/4(Re)
  [Re] -> Fy Relaxation/4(Re)
  [sig_x] -> My Relaxation/5(sig_x)
  [Re] -> My Relaxation/4(Re)
  [sig_x] -> Fx Relaxation/5(sig_x)
  Magic Tire Const Input/11(sig_y) -> [sig_y]
  Magic Tire Const Input/10(sig_x) -> [sig_x]
  [Omega] -> Fx Relaxation/1(omega)
  [Vx] -> Fx Relaxation/2(Vx)
  Fy Relaxation/1(y) -> [Fy], LateralForce/1
  Magic Tire Const Input/12(a) -> a/1
  Magic Tire Const Input/13(b) -> b/1
  Magic Tire Const Input/5(My) -> My Relaxation/3(My)
  Vy/1 -> Magic Tire Const Input/3(Vy), [Vy]
  Vx/1 -> Magic Tire Const Input/2(Vx), [Vx]
  My Relaxation/1(y) -> RollingResistance/1
  Fx Relaxation/1(y) -> [Fx], LongitudinalForce/1
  Magic Tire Const Input/7(Re) -> EffectiveRadius/1, [Re]
  Magic Tire Const Input/2(Fy) -> Fy Relaxation/3(Fy)
  Magic Tire Const Input/9(Alpha) -> SlipAngle/1
  Magic Tire Const Input/8(Kappa) -> SlipRatio/1
  Magic Tire Const Input/6(Mz) -> AligningTorque/1
  Magic Tire Const Input/4(Mx) -> OverturningTorque/1
  Deflection/1 -> Magic Tire Const Input/8(rhoz)
  ScaleFactors/1 -> Magic Tire Const Input/7(ScaleFactors)
  TirePrs/1 -> Magic Tire Const Input/6(TirePrs)
  Camber/1 -> Magic Tire Const Input/5(Gamma)
  YawRate/1 -> Magic Tire Const Input/4(psidot)
  Omega/1 -> [Omega], Magic Tire Const Input/1(Omega)
  Magic Tire Const Input/3(FzTire) -> FzTire/1

== system vehicle_motion_model_final_temp/Two-Axle Vehicle/Vehicle Body/Vehicle Body 6DOF/Vehicle Body 6DOF/6 DOF Generic Vehicle Body/SignalCollection/Angle Wrap/None ==
  u : Inport
  y : Outport  VectorParamsAs1DForOutWhenUnconnected=off
  wires:
  u/1 -> y/1

== system vehicle_motion_model_final_temp/Two-Axle Vehicle/Vehicle Body/Vehicle Body 6DOF/Vehicle Body 6DOF/Moment Calc/Hitch moments from forces/hitch geometry parameters/hitch active ==
  Constant : Constant  Value=dh
  Constant1 : Constant  Value=hh
  Constant2 : Constant  Value=hl
  dh_out : Outport  VectorParamsAs1DForOutWhenUnconnected=off
  hh_out : Outport  Port=2  VectorParamsAs1DForOutWhenUnconnected=off
  hl_out : Outport  Port=3  VectorParamsAs1DForOutWhenUnconnected=off
  wires:
  Constant/1 -> dh_out/1
  Constant1/1 -> hh_out/1
  Constant2/1 -> hl_out/1

== system vehicle_motion_model_final_temp/Two-Axle Vehicle/Vehicle Body/Vehicle Body 6DOF/Vehicle Body 6DOF/Moment Calc/Hitch moments from forces/hitch geometry parameters/hitch inactive ==
  Ground : Ground
  dh_out : Outport  Unit=m  PortDimensions=1  VectorParamsAs1DForOutWhenUnconnected=off
  hh_out : Outport  Port=2  Unit=m  PortDimensions=1  VectorParamsAs1DForOutWhenUnconnected=off
  hl_out : Outport  Port=3  Unit=m  PortDimensions=1  VectorParamsAs1DForOutWhenUnconnected=off
  wires:
  Ground/1 -> hl_out/1, hh_out/1, dh_out/1

== system vehicle_motion_model_final_temp/Two-Axle Vehicle/Wheels and Tires/Wheels and Tires/Tires/MF Tires/Combined Slip Wheel 2DOF/Magic Tire Const Input/Fx Relaxation ==
  omega : Inport
  Vx : Inport  Port=2
  Fx : Inport  Port=3
  Re : Inport  Port=4
  sig_x : Inport  Port=5
  Abs : Abs  ZeroCross=off
  Add : Sum  Inputs=+-
  Add1 : Sum  Inputs=+-
  Integrator : Integrator  UpperSaturationLimit=10e3  LowerSaturationLimit=-10e3  ZeroCross=off
  Product1 : Product  Inputs=**
  Product2 : Product  Inputs=**
  Product3 : Product  Inputs=*/
  Saturation : Saturate  UpperLimit=inf  LowerLimit=FxRelFreqLwrLim  ZeroCross=off
  Saturation1 : Saturate  UpperLimit=inf  LowerLimit=1e-2  ZeroCross=off
  y : Outport  VectorParamsAs1DForOutWhenUnconnected=off
  wires:
  Add1/1 -> Abs/1
  Add/1 -> Product1/2
  Integrator/1 -> y/1, Add/2
  Product1/1 -> Integrator/1
  Product3/1 -> Saturation/1
  Saturation/1 -> Product1/1
  Fx/1 -> Add/1
  Vx/1 -> Add1/1
  Abs/1 -> Product3/1
  Saturation1/1 -> Product3/2
  sig_x/1 -> Saturation1/1
  omega/1 -> Product2/1
  Re/1 -> Product2/2
  Product2/1 -> Add1/2

== system vehicle_motion_model_final_temp/Two-Axle Vehicle/Wheels and Tires/Wheels and Tires/Tires/MF Tires/Combined Slip Wheel 2DOF/Magic Tire Const Input/Fy Relaxation ==
  omega : Inport
  Vy : Inport  Port=2
  Fy : Inport  Port=3
  Re : Inport  Port=4
  sig_y : Inport  Port=5
  Abs : Abs  ZeroCross=off
  Add : Sum  Inputs=+-
  Add1 : Sum  Inputs=+-
  Integrator : Integrator  UpperSaturationLimit=10e3  LowerSaturationLimit=-10e3  ZeroCross=off
  Product1 : Product  Inputs=**
  Product2 : Product  Inputs=**
  Product3 : Product  Inputs=*/
  Saturation : Saturate  UpperLimit=inf  LowerLimit=FyRelFreqLwrLim  ZeroCross=off
  Saturation1 : Saturate  UpperLimit=inf  LowerLimit=1e-2  ZeroCross=off
  y : Outport  VectorParamsAs1DForOutWhenUnconnected=off
  wires:
  Product3/1 -> Saturation/1
  Fy/1 -> Add/1
  Add/1 -> Product1/2
  Product1/1 -> Integrator/1
  Saturation/1 -> Product1/1
  Vy/1 -> Add1/1
  Integrator/1 -> Add/2, y/1
  Product2/1 -> Add1/2
  Re/1 -> Product2/2
  omega/1 -> Product2/1
  Add1/1 -> Abs/1
  sig_y/1 -> Saturation1/1
  Saturation1/1 -> Product3/2
  Abs/1 -> Product3/1

== system vehicle_motion_model_final_temp/Two-Axle Vehicle/Wheels and Tires/Wheels and Tires/Tires/MF Tires/Combined Slip Wheel 2DOF/Magic Tire Const Input/My Relaxation ==
  omega : Inport
  Vx : Inport  Port=2
  My : Inport  Port=3
  Re : Inport  Port=4
  sig_x : Inport  Port=5
  Abs : Abs  ZeroCross=off
  Add : Sum  Inputs=+-
  Add1 : Sum  Inputs=+-
  Integrator : Integrator  UpperSaturationLimit=10e3  LowerSaturationLimit=-10e3  ZeroCross=off
  Product1 : Product  Inputs=**
  Product2 : Product  Inputs=**
  Product3 : Product  Inputs=*/
  Saturation : Saturate  UpperLimit=inf  LowerLimit=MyRelFreqLwrLim  ZeroCross=off
  Saturation1 : Saturate  UpperLimit=inf  LowerLimit=1e-2  ZeroCross=off
  y : Outport  VectorParamsAs1DForOutWhenUnconnected=off
  wires:
  Product3/1 -> Saturation/1
  Saturation/1 -> Product1/1
  Product2/1 -> Add1/2
  Vx/1 -> Add1/1
  Re/1 -> Product2/2
  omega/1 -> Product2/1
  My/1 -> Add/1
  Product1/1 -> Integrator/1
  Add/1 -> Product1/2
  Add1/1 -> Abs/1
  sig_x/1 -> Saturation1/1
  Saturation1/1 -> Product3/2
  Integrator/1 -> y/1, Add/2
  Abs/1 -> Product3/1

== matlab function vehicle_motion_model_final_temp/Calc errors3/To angles ==
  data: qat input; ang output
function ang = fcn(qat)
%#codegen
    q0 = qat(1);
    q1 = qat(2);
    q2 = qat(3);
    q3 = qat(4);
    phi = atan2(2*(q2*q3 + q0*q1), (q0^2 - q1^2 - q2^2 - q3^2));
    theta = asin(-2*(q1*q3 - q0*q2));
    psi = atan2(2*(q1*q2 +q0*q3), (q0^2 + q1^2 - q2^2 - q3^2));
    ang = [phi; theta; psi];
end

== matlab function vehicle_motion_model_final_temp/Prediction step (BINS)/Prediction ==
  data: x_ input; x output; P output; P_ input; dT input; BINS_output input
function [x, P] = prediction(x_, P_, dT, BINS_output)
% do prediction step

    sigma_IMU_a = 0.0001;
    sigma_IMU_w = 0.0001;
    sigma_IMU_ab = 0;
    sigma_IMU_wb = 0;
    Q = eye(12);
    Q(1:3, 1:3) = sigma_IMU_a * sigma_IMU_a * Q(1:3, 1:3)*dT*dT;
    Q(4:6, 4:6) = sigma_IMU_w * sigma_IMU_w * Q(4:6, 4:6)*dT*dT;
    Q(7:9, 7:9) = sigma_IMU_ab * sigma_IMU_ab * Q(7:9, 7:9)*dT;
    Q(10:12, 10:12) = sigma_IMU_wb * sigma_IMU_wb * Q(10:12, 10:12)*dT;
    L_jac = zeros(18, 12);
    L_jac(4:15, :) = eye(12);

    % Update nominal state with IMU inputs
    x = F_func(x_, dT, BINS_output);
    % Linearize Motion Model and compute Jacobians (for the error state)
    F_jac = DF_func(x_, dT, BINS_output);
    % Propagate uncertainty
    P = F_jac*P_*transpose(F_jac) + L_jac*Q*transpose(L_jac);
end

== matlab function vehicle_motion_model_final_temp/BINS kinematics Euler/calc rotation matrix ==
  data: ang input; DCM_calc output
function DCM_calc = fcn(ang)
    DCM_calc = DCM_calc_from_angles(ang);
end

== matlab function vehicle_motion_model_final_temp/Two-Axle Vehicle/Vehicle Body/Vehicle Body 6DOF/Vehicle Body 6DOF/vehdyncginert ==
  data: m parameter size=1; Mbar output size=1; z1m parameter size=1; z2m parameter size=1; z3m parameter size=1; z4m parameter size=1; z5m parameter size=1; z6m parameter size=1; z7m parameter size=1; z1R parameter size=[1,3]; z2R parameter size=[1,3]; z3R parameter size=[1,3]; z4R parameter size=[1,3]; z5R parameter size=[1,3]; z6R parameter size=[1,3]; Iveh parameter size=[3,3]; z1I parameter size=[3,3]; z2I parameter size=[3,3]; z3I parameter size=[3,3]; z4I parameter size=[3,3]; z5I parameter size=[3,3]; z6I parameter size=[3,3]; z7I parameter size=[3,3]; Ibar output size=[3,3]; Rbar output; z7R parameter size=[1,3]; Xbar output; Wbar output; a parameter size=1; b parameter size=1; h parameter size=1; w parameter size=2; d parameter; HPbar output size=[3,4]
function [Mbar,Ibar,Rbar,Xbar,Wbar,HPbar] = inert(m, z1m, z2m, z3m, z4m, z5m, z6m, z7m,z1R, z2R, z3R, z4R, z5R, z6R, Iveh, z1I, z2I, z3I, z4I, z5I, z6I, z7I, z7R, a, b, h, w, d)%#codegen
coder.allowpcode('plain')
[Rbar,Mbar,Ibar,Xbar,Wbar,HPbar]= vehdyncginerthp(m, z1m, z2m, z3m, z4m, z5m, z6m, z7m,z1R, z2R, z3R, z4R, z5R, z6R, Iveh, z1I, z2I, z3I, z4I, z5I, z6I, z7I, z7R, a, b, h, w, d);
end

== matlab function vehicle_motion_model_final_temp/Vehicle Selector/calc rotation matrix1 ==
  data: ang input; DCM_calc output
function DCM_calc = fcn(ang)
    DCM_calc = DCM_calc_from_angles(ang);
end
